simulink model "Main_C0_C3"  (R2023a)
settings: Solver=ode15s  StartTime=0.0  StopTime=1  RelTol=1e-3
model workspace (MAT data in the model file):
  C_IVD = 0.05
  E_IVD1 = 2.1
  E_IVD2 = 2.2
  E_IVD3 = 1.1
  E_IVD4 = 1.7
  E_IVD5 = 3.2
  IVD1 : object (value not decoded)
  IVD2 : object (value not decoded)
  IVD3 : object (value not decoded)
  IVD4 : object (value not decoded)
  IVD5 : object (value not decoded)
  eo_color = [1 0 0]
  io_color = [0 1 0]
  longissimus_color = [1 0 1]
  multifidus_color = [0 1 1]
  muscle_radius = 1
  psoas_color = [0 0 1]
  ra_color = [1 1 0.5]
symbols that are objects in the model workspace (value not decoded): IVD1, IVD2, IVD3, IVD4, IVD5
undefined symbols (not defined in the file or in its folder): AbdFlex, E_TLFflex, IAP_activation_AbdFlex, IAP_Pa, LeftAbdominalMuscleForce, LeftBackMuscleForce, LeftTransverse1MuscleForce, LeftTransverse2MuscleForce, RightAbdominalMuscleForce, RightBackMuscleForce, RightTransverse1MuscleForce, RightTransverse2MuscleForce, TLFflex2, X, Y, Z
libraries: nesl_utility x1235, sm_lib x960, fl_lib x6, simulink_extras x2
(part 7 of 37)

== system Main_C0_C3/TLF Flex ==
  note: F1 - F5 = connectors
      | F6 = right holder
      | F7 = left holder
      | F8 - F10 = right latissimus
      | F11 - F13 = left latissimus
  note: Note: You CAN'T use Fast Restart with Flexible Bodies !
      | They need to be compiled every run, because of E_flex.
  In1 : Inport
  In2 : Inport  Port=2
  Conn L1 : sm_lib/Body Elements/File Solid  ExtGeomFileName=C:\Users\siril\OneDrive\Desktop\TIM-Control\Matlab\Simscape models\Reduced Order Model\CAD\model without nucleus\TLF\L1-conn.step  UnitType=FromFile  ExtGeomFileUnits=m  StepReaderType=HEX  ExportConvexHullGeometry=off  InertiaType=Custom  Mass=1  MassUnits=g  CenterOfMass=[0 0 0]  CenterOfMassUnits=m  MomentsOfInertia=[1 1 1]  MomentsOfInertiaUnits=kg*m^2  ProductsOfInertia=[0 0 0]  ProductsOfInertiaUnits=kg*m^2  BasedOnType=DensityFromFile  Density=1000  DensityUnits=kg/m^3  DoExposeReferenceFrame=off  SerializedFrames=<Frames><Frame><Id>Frame1</Id><Value><Name>to L1_Muscles</Name><Origin><Source>GeometricFeature</Source><FeatureName>point 120</FeatureName></Origin><PrimaryAxis><DefinedDirection>+Z</DefinedDirection><Source>ReferenceFrame</Source><SourceDirection>+Z</SourceDirection><FeatureName></FeatureName></PrimaryAxis><SecondaryAxis><DefinedDirection>+X</DefinedDirection><Source>ReferenceFrame</Source><SourceDirection>+X</SourceDirection><FeatureName></FeatureName></SecondaryAxis></Value></Frame><Frame><Id>Frame2</Id><Value><Name>to TLF</Name><Origin><Source>GeometricFeature</Source><FeatureName>planar surface 1</FeatureName></Origin><PrimaryAxis><DefinedDirection>+Z</DefinedDirection><Source>ReferenceFrame</Source><SourceDirection>+Z</SourceDirection><FeatureName></FeatureName></PrimaryAxis><SecondaryAxis><DefinedDirection>+X</DefinedDirection><Source>ReferenceFrame</Source><SourceDirection>+X</SourceDirection><FeatureName></FeatureName></SecondaryAxis></Value></Frame></Frames>  GraphicType=None  MarkerShape=Sphere  MarkerSize=10  GraphicVisPropType=SimpleVisualProperties  GraphicDiffuseColor=[0.5 0.5 0.5]  GraphicSpecularColor=[0.5 0.5 0.5 1.0]  GraphicAmbientColor=[0.15 0.15 0.15 1.0]  GraphicEmissiveColor=[0.0 0.0 0.0 1.0]  GraphicShininess=75  GraphicOpacity=0.5
  Conn L2 : sm_lib/Body Elements/File Solid  ExtGeomFileName=C:\Users\siril\OneDrive\Desktop\TIM-Control\Matlab\Simscape models\Reduced Order Model\CAD\model without nucleus\TLF\L2-conn.step  UnitType=FromFile  ExtGeomFileUnits=m  StepReaderType=HEX  ExportConvexHullGeometry=off  InertiaType=Custom  Mass=1  MassUnits=g  CenterOfMass=[0 0 0]  CenterOfMassUnits=m  MomentsOfInertia=[1 1 1]  MomentsOfInertiaUnits=kg*m^2  ProductsOfInertia=[0 0 0]  ProductsOfInertiaUnits=kg*m^2  BasedOnType=DensityFromFile  Density=1000  DensityUnits=kg/m^3  DoExposeReferenceFrame=off  SerializedFrames=<Frames><Frame><Id>Frame1</Id><Value><Name>to Muscles L2</Name><Origin><Source>GeometricFeature</Source><FeatureName>point 118</FeatureName></Origin><PrimaryAxis><DefinedDirection>+Z</DefinedDirection><Source>ReferenceFrame</Source><SourceDirection>+Z</SourceDirection><FeatureName></FeatureName></PrimaryAxis><SecondaryAxis><DefinedDirection>+X</DefinedDirection><Source>ReferenceFrame</Source><SourceDirection>+X</SourceDirection><FeatureName></FeatureName></SecondaryAxis></Value></Frame><Frame><Id>Frame2</Id><Value><Name>to TLF</Name><Origin><Source>GeometricFeature</Source><FeatureName>planar surface 1</FeatureName></Origin><PrimaryAxis><DefinedDirection>+Z</DefinedDirection><Source>ReferenceFrame</Source><SourceDirection>+Z</SourceDirection><FeatureName></FeatureName></PrimaryAxis><SecondaryAxis><DefinedDirection>+X</DefinedDirection><Source>ReferenceFrame</Source><SourceDirection>+X</SourceDirection><FeatureName></FeatureName></SecondaryAxis></Value></Frame></Frames>  GraphicType=None  MarkerShape=Sphere  MarkerSize=10  GraphicVisPropType=SimpleVisualProperties  GraphicDiffuseColor=[0.5 0.5 0.5]  GraphicSpecularColor=[0.5 0.5 0.5 1.0]  GraphicAmbientColor=[0.15 0.15 0.15 1.0]  GraphicEmissiveColor=[0.0 0.0 0.0 1.0]  GraphicShininess=75  GraphicOpacity=0.5
  Conn L3 : sm_lib/Body Elements/File Solid  ExtGeomFileName=C:\Users\siril\OneDrive\Desktop\TIM-Control\Matlab\Simscape models\Reduced Order Model\CAD\model without nucleus\TLF\L3-conn.step  UnitType=FromFile  ExtGeomFileUnits=m  StepReaderType=HEX  ExportConvexHullGeometry=off  InertiaType=Custom  Mass=1  MassUnits=g  CenterOfMass=[0 0 0]  CenterOfMassUnits=m  MomentsOfInertia=[1 1 1]  MomentsOfInertiaUnits=kg*m^2  ProductsOfInertia=[0 0 0]  ProductsOfInertiaUnits=kg*m^2  BasedOnType=DensityFromFile  Density=1000  DensityUnits=kg/m^3  DoExposeReferenceFrame=off  SerializedFrames=<Frames><Frame><Id>Frame1</Id><Value><Name>to Muscles L3</Name><Origin><Source>GeometricFeature</Source><FeatureName>point 147</FeatureName></Origin><PrimaryAxis><DefinedDirection>+Z</DefinedDirection><Source>ReferenceFrame</Source><SourceDirection>+Z</SourceDirection><FeatureName></FeatureName></PrimaryAxis><SecondaryAxis><DefinedDirection>+X</DefinedDirection><Source>ReferenceFrame</Source><SourceDirection>+X</SourceDirection><FeatureName></FeatureName></SecondaryAxis></Value></Frame><Frame><Id>Frame2</Id><Value><Name>to TLF</Name><Origin><Source>GeometricFeature</Source><FeatureName>planar surface 1</FeatureName></Origin><PrimaryAxis><DefinedDirection>+Z</DefinedDirection><Source>ReferenceFrame</Source><SourceDirection>+Z</SourceDirection><FeatureName></FeatureName></PrimaryAxis><SecondaryAxis><DefinedDirection>+X</DefinedDirection><Source>ReferenceFrame</Source><SourceDirection>+X</SourceDirection><FeatureName></FeatureName></SecondaryAxis></Value></Frame></Frames>  GraphicType=None  MarkerShape=Sphere  MarkerSize=10  GraphicVisPropType=SimpleVisualProperties  GraphicDiffuseColor=[0.5 0.5 0.5]  GraphicSpecularColor=[0.5 0.5 0.5 1.0]  GraphicAmbientColor=[0.15 0.15 0.15 1.0]  GraphicEmissiveColor=[0.0 0.0 0.0 1.0]  GraphicShininess=75  GraphicOpacity=0.5
  Conn L4 : sm_lib/Body Elements/File Solid  ExtGeomFileName=C:\Users\siril\OneDrive\Desktop\TIM-Control\Matlab\Simscape models\Reduced Order Model\CAD\model without nucleus\TLF\L4-conn.step  UnitType=FromFile  ExtGeomFileUnits=m  StepReaderType=HEX  ExportConvexHullGeometry=off  InertiaType=Custom  Mass=1  MassUnits=g  CenterOfMass=[0 0 0]  CenterOfMassUnits=m  MomentsOfInertia=[1 1 1]  MomentsOfInertiaUnits=kg*m^2  ProductsOfInertia=[0 0 0]  ProductsOfInertiaUnits=kg*m^2  BasedOnType=DensityFromFile  Density=1000  DensityUnits=kg/m^3  DoExposeReferenceFrame=off  SerializedFrames=<Frames><Frame><Id>Frame1</Id><Value><Name>to Muscles L4</Name><Origin><Source>GeometricFeature</Source><FeatureName>point 96</FeatureName></Origin><PrimaryAxis><DefinedDirection>+Z</DefinedDirection><Source>ReferenceFrame</Source><SourceDirection>+Z</SourceDirection><FeatureName></FeatureName></PrimaryAxis><SecondaryAxis><DefinedDirection>+X</DefinedDirection><Source>ReferenceFrame</Source><SourceDirection>+X</SourceDirection><FeatureName></FeatureName></SecondaryAxis></Value></Frame><Frame><Id>Frame2</Id><Value><Name>to TLF</Name><Origin><Source>GeometricFeature</Source><FeatureName>planar surface 3</FeatureName></Origin><PrimaryAxis><DefinedDirection>+Z</DefinedDirection><Source>ReferenceFrame</Source><SourceDirection>+Z</SourceDirection><FeatureName></FeatureName></PrimaryAxis><SecondaryAxis><DefinedDirection>+X</DefinedDirection><Source>ReferenceFrame</Source><SourceDirection>+X</SourceDirection><FeatureName></FeatureName></SecondaryAxis></Value></Frame></Frames>  GraphicType=None  MarkerShape=Sphere  MarkerSize=10  GraphicVisPropType=SimpleVisualProperties  GraphicDiffuseColor=[0.5 0.5 0.5]  GraphicSpecularColor=[0.5 0.5 0.5 1.0]  GraphicAmbientColor=[0.15 0.15 0.15 1.0]  GraphicEmissiveColor=[0.0 0.0 0.0 1.0]  GraphicShininess=75  GraphicOpacity=0.5
  Conn L5 : sm_lib/Body Elements/File Solid  ExtGeomFileName=C:\Users\siril\OneDrive\Desktop\TIM-Control\Matlab\Simscape models\Reduced Order Model\CAD\model without nucleus\TLF\L5-conn.step  UnitType=FromFile  ExtGeomFileUnits=m  StepReaderType=HEX  ExportConvexHullGeometry=off  InertiaType=Custom  Mass=1  MassUnits=g  CenterOfMass=[0 0 0]  CenterOfMassUnits=m  MomentsOfInertia=[1 1 1]  MomentsOfInertiaUnits=kg*m^2  ProductsOfInertia=[0 0 0]  ProductsOfInertiaUnits=kg*m^2  BasedOnType=DensityFromFile  Density=1000  DensityUnits=kg/m^3  DoExposeReferenceFrame=off  SerializedFrames=<Frames><Frame><Id>Frame1</Id><Value><Name>to Muscles L5</Name><Origin><Source>GeometricFeature</Source><FeatureName>point 125</FeatureName></Origin><PrimaryAxis><DefinedDirection>+Z</DefinedDirection><Source>ReferenceFrame</Source><SourceDirection>+Z</SourceDirection><FeatureName></FeatureName></PrimaryAxis><SecondaryAxis><DefinedDirection>+X</DefinedDirection><Source>ReferenceFrame</Source><SourceDirection>+X</SourceDirection><FeatureName></FeatureName></SecondaryAxis></Value></Frame><Frame><Id>Frame2</Id><Value><Name>to TLF</Name><Origin><Source>GeometricFeature</Source><FeatureName>planar surface 1</FeatureName></Origin><PrimaryAxis><DefinedDirection>+Z</DefinedDirection><Source>ReferenceFrame</Source><SourceDirection>+Z</SourceDirection><FeatureName></FeatureName></PrimaryAxis><SecondaryAxis><DefinedDirection>+X</DefinedDirection><Source>ReferenceFrame</Source><SourceDirection>+X</SourceDirection><FeatureName></FeatureName></SecondaryAxis></Value></Frame></Frames>  GraphicType=None  MarkerShape=Sphere  MarkerSize=10  GraphicVisPropType=SimpleVisualProperties  GraphicDiffuseColor=[0.5 0.5 0.5]  GraphicSpecularColor=[0.5 0.5 0.5 1.0]  GraphicAmbientColor=[0.15 0.15 0.15 1.0]  GraphicEmissiveColor=[0.0 0.0 0.0 1.0]  GraphicShininess=75  GraphicOpacity=0.5
  Holder left : sm_lib/Body Elements/File Solid  ExtGeomFileName=C:\Users\siril\OneDrive\Desktop\TIM-Control\Matlab\Simscape models\Reduced Order Model\CAD\model without nucleus\TLF\Holder_left.step  UnitType=FromFile  ExtGeomFileUnits=m  StepReaderType=HEX  ExportConvexHullGeometry=off  InertiaType=Custom  Mass=1  MassUnits=g  CenterOfMass=[0 0 0]  CenterOfMassUnits=m  MomentsOfInertia=[1 1 1]  MomentsOfInertiaUnits=kg*m^2  ProductsOfInertia=[0 0 0]  ProductsOfInertiaUnits=kg*m^2  BasedOnType=DensityFromFile  Density=1000  DensityUnits=kg/m^3  DoExposeReferenceFrame=on  SerializedFrames=<Frames><Frame><Id>Frame1</Id><Value><Name>F1</Name><Origin><Source>GeometricFeature</Source><FeatureName>general surface 1</FeatureName></Origin><PrimaryAxis><DefinedDirection>+Z</DefinedDirection><Source>ReferenceFrame</Source><SourceDirection>+Z</SourceDirection><FeatureName></FeatureName></PrimaryAxis><SecondaryAxis><DefinedDirection>+X</DefinedDirection><Source>ReferenceFrame</Source><SourceDirection>+X</SourceDirection><FeatureName></FeatureName></SecondaryAxis></Value></Frame></Frames>  GraphicType=None  MarkerShape=Sphere  MarkerSize=10  GraphicVisPropType=SimpleVisualProperties  GraphicDiffuseColor=[0.5 0.5 0.5]  GraphicSpecularColor=[0.5 0.5 0.5 1.0]  GraphicAmbientColor=[0.15 0.15 0.15 1.0]  GraphicEmissiveColor=[0.0 0.0 0.0 1.0]  GraphicShininess=75  GraphicOpacity=1.0
  Holder right : sm_lib/Body Elements/File Solid  ExtGeomFileName=C:\Users\siril\OneDrive\Desktop\TIM-Control\Matlab\Simscape models\Reduced Order Model\CAD\model without nucleus\TLF\Holder_right.step  UnitType=FromFile  ExtGeomFileUnits=m  StepReaderType=HEX  ExportConvexHullGeometry=off  InertiaType=Custom  Mass=1  MassUnits=g  CenterOfMass=[0 0 0]  CenterOfMassUnits=m  MomentsOfInertia=[1 1 1]  MomentsOfInertiaUnits=kg*m^2  ProductsOfInertia=[0 0 0]  ProductsOfInertiaUnits=kg*m^2  BasedOnType=DensityFromFile  Density=1000  DensityUnits=kg/m^3  DoExposeReferenceFrame=on  SerializedFrames=<Frames><Frame><Id>Frame1</Id><Value><Name>F1</Name><Origin><Source>GeometricFeature</Source><FeatureName>general surface 1</FeatureName></Origin><PrimaryAxis><DefinedDirection>+Z</DefinedDirection><Source>ReferenceFrame</Source><SourceDirection>+Z</SourceDirection><FeatureName></FeatureName></PrimaryAxis><SecondaryAxis><DefinedDirection>+X</DefinedDirection><Source>ReferenceFrame</Source><SourceDirection>+X</SourceDirection><FeatureName></FeatureName></SecondaryAxis></Value></Frame></Frames>  GraphicType=None  MarkerShape=Sphere  MarkerSize=10  GraphicVisPropType=SimpleVisualProperties  GraphicDiffuseColor=[0.5 0.5 0.5]  GraphicSpecularColor=[0.5 0.5 0.5 1.0]  GraphicAmbientColor=[0.15 0.15 0.15 1.0]  GraphicEmissiveColor=[0.0 0.0 0.0 1.0]  GraphicShininess=75  GraphicOpacity=1.0
  Latissimus Dorsi : Subsystem
  TLF_Flex : sm_lib/Body Elements/Flexible Bodies/Reduced Order Flexible Solid  GraphicAmbientColor=[0.15 0.15 0.15 1.0]  GraphicDiffuseColor=[0.07451 0.6235 1]  DampingType=Proportional  GraphicEmissiveColor=[0.0 0.0 0.0 1.0]  GraphicFacetVertexIndices=TLFflex2.GraphicFacetVertexIndices  InterfaceFrameOrientations=TLFflex2.InterfaceFrameOrientations  GraphicType=DeformedGeometry  MassMatrix=TLFflex2.MassMatrix  NumRetainedModes=1  NumberOfInterfaceFrames=13  GraphicOpacity=0.2  GraphicReconstructionMatrix=TLFflex2.GraphicReconstructionMatrix  ReductionType=None  InterfaceFrameOrigins=TLFflex2.InterfaceFrameOrigins  GraphicShininess=75  GraphicSpecularColor=[0.5 0.5 0.5 1.0]  StiffnessMatrix=TLFflex2.StiffnessMatrix * E_TLFflex  GeomUnitType=FromFile  GraphicVertexCoordinates=TLFflex2.GraphicVertexCoordinates  VisRecursionLimit=3  GraphicVisPropType=SimpleVisualProperties  LengthUnit=m  MassUnit=kg  TimeUnit=s  UnitSystemType=SI  ProportionalDampingAlpha=0  ProportionalDampingBeta=0.05  UniformModalDampingRatio=0.01  DampingMatrix=[]
  Weld Joint11 : sm_lib/Joints/Weld Joint  JointMode=Normal  SenseConstraintForce=off  SenseConstraintForceX=off  SenseConstraintForceY=off  SenseConstraintForceZ=off  SenseConstraintTorque=off  SenseConstraintTorqueX=off  SenseConstraintTorqueY=off  SenseConstraintTorqueZ=off  SenseTotalForce=off  SenseTotalForceX=off  SenseTotalForceY=off  SenseTotalForceZ=off  SenseTotalTorque=off  SenseTotalTorqueX=off  SenseTotalTorqueY=off  SenseTotalTorqueZ=off  CompositeWrenchDir=FollowerOnBase  CompositeWrenchFrame=BaseFrame
  Weld Joint12 : sm_lib/Joints/Weld Joint  JointMode=Normal  SenseConstraintForce=off  SenseConstraintForceX=off  SenseConstraintForceY=off  SenseConstraintForceZ=off  SenseConstraintTorque=off  SenseConstraintTorqueX=off  SenseConstraintTorqueY=off  SenseConstraintTorqueZ=off  SenseTotalForce=off  SenseTotalForceX=off  SenseTotalForceY=off  SenseTotalForceZ=off  SenseTotalTorque=off  SenseTotalTorqueX=off  SenseTotalTorqueY=off  SenseTotalTorqueZ=off  CompositeWrenchDir=FollowerOnBase  CompositeWrenchFrame=BaseFrame
  Conn1 : PMIOPort  Side=Left
  Conn2 : PMIOPort  Port=2  Side=Left
  Conn3 : PMIOPort  Port=3  Side=Left
  Conn4 : PMIOPort  Port=4  Side=Left
  Conn5 : PMIOPort  Port=5  Side=Left
  Conn6 : PMIOPort  Port=6  Side=Right
  Wrap1 : PMIOPort  Port=7  Side=Right
  Wrap2 : PMIOPort  Port=8  Side=Right
  Conn9 : PMIOPort  Port=9  Side=Left
  Conn10 : PMIOPort  Port=10  Side=Right
  Conn11 : PMIOPort  Port=11  Side=Left
  Conn12 : PMIOPort  Port=12  Side=Left
  Conn13 : PMIOPort  Port=13  Side=Right
  Wrap3 : PMIOPort  Port=14  Side=Right
  Conn15 : PMIOPort  Port=15  Side=Left
  Wrap4 : PMIOPort  Port=16  Side=Right
  Conn17 : PMIOPort  Port=17  Side=Left
  Wrap5 : PMIOPort  Port=18  Side=Right
  wires:
  In1/1 -> Latissimus Dorsi/1(In1)
  In2/1 -> Latissimus Dorsi/2(In2)
  connections:
  Latissimus Dorsi/LConn5 -- Conn17/RConn1
  Latissimus Dorsi/RConn10 -- Wrap5/RConn1
  Latissimus Dorsi/LConn6 -- Conn9/RConn1
  Conn5/RConn1 -- Conn L2/LConn1
  Conn13/RConn1 -- Latissimus Dorsi/RConn1
  Latissimus Dorsi/LConn4 -- Conn15/RConn1
  Conn4/RConn1 -- Conn L5/LConn1
  Conn1/RConn1 -- Conn L4/LConn1
  Latissimus Dorsi/RConn6 -- Wrap2/RConn1
  Latissimus Dorsi/RConn8 -- Wrap3/RConn1
  Latissimus Dorsi/RConn7 -- Conn10/RConn1
  Conn6/RConn1 -- Latissimus Dorsi/RConn11
  Latissimus Dorsi/RConn5 -- Wrap1/RConn1
  Weld Joint11/RConn1 -- TLF_Flex/RConn3
  Holder right/LConn1 -- Weld Joint11/LConn1
  Conn2/RConn1 -- Conn L3/LConn1
  Conn L4/RConn1 -- TLF_Flex/RConn2
  Holder left/LConn1 -- Weld Joint12/LConn1
  Weld Joint12/RConn1 -- TLF_Flex/LConn4
  Latissimus Dorsi/LConn7 -- Conn11/RConn1
  Latissimus Dorsi/RConn9 -- Wrap4/RConn1
  Latissimus Dorsi/RConn2 -- TLF_Flex/LConn5
  Latissimus Dorsi/LConn1 -- TLF_Flex/RConn4
  Latissimus Dorsi/LConn3 -- TLF_Flex/RConn6
  Latissimus Dorsi/RConn4 -- TLF_Flex/LConn7
  Conn3/RConn1 -- Conn L1/LConn1
  Holder right/RConn1 -- Conn12/RConn1 -- Holder left/RConn1
  Conn L1/RConn1 -- TLF_Flex/LConn1
  Latissimus Dorsi/RConn3 -- TLF_Flex/LConn6
  Conn L3/RConn1 -- TLF_Flex/LConn2
  Latissimus Dorsi/LConn2 -- TLF_Flex/RConn5
  Conn L5/RConn1 -- TLF_Flex/LConn3
  Conn L2/RConn1 -- TLF_Flex/RConn1

== system Main_C0_C3/Interspinous Ligaments/ISL Visualization ==
  Ligament1 : Subsystem
  Ligament2 : Subsystem
  Ligament3 : Subsystem
  Ligament4 : Subsystem
  Ligament5 : Subsystem
  MuscleEnd2 : PMIOPort  Side=Right
  MuscleEnd1 : PMIOPort  Port=2  Side=Right
  MuscleEnd3 : PMIOPort  Port=3  Side=Right
  MuscleEnd4 : PMIOPort  Port=4  Side=Right
  MuscleEnd5 : PMIOPort  Port=5  Side=Right
  MuscleEnd6 : PMIOPort  Port=6  Side=Right
  MuscleEnd7 : PMIOPort  Port=7  Side=Right
  MuscleEnd8 : PMIOPort  Port=8  Side=Right
  MuscleEnd9 : PMIOPort  Port=9  Side=Right
  MuscleEnd10 : PMIOPort  Port=10  Side=Right
  R : PMIOPort  Port=11  Side=Left
  connections:
  Ligament2/RConn2 -- MuscleEnd6/RConn1
  Ligament4/RConn2 -- MuscleEnd1/RConn1
  Ligament5/RConn1 -- MuscleEnd3/RConn1
  Ligament2/RConn1 -- MuscleEnd9/RConn1
  Ligament5/RConn2 -- MuscleEnd2/RConn1
  Ligament1/RConn2 -- MuscleEnd10/RConn1
  Ligament3/RConn1 -- MuscleEnd7/RConn1
  Ligament3/RConn2 -- MuscleEnd5/RConn1
  Ligament4/RConn3 -- Ligament3/RConn3 -- Ligament2/RConn3 -- R/RConn1 -- Ligament1/RConn3 -- Ligament5/RConn3
  Ligament4/RConn1 -- MuscleEnd4/RConn1
  Ligament1/RConn1 -- MuscleEnd8/RConn1

== system Main_C0_C3/Interspinous Ligaments/Visualization ==
  Belt-Cable Properties{1..4,55} (5 alike) : sm_lib/Belts and Cables/Belt-Cable Properties  DrumBeltCableAlignment=Unrestricted  GraphicType=PitchLine  GraphicVisPropType=SimpleVisualProperties  GraphicDiffuseColor=[1 0 1]  GraphicSpecularColor=[0.5 0.5 0.5 1.0]  GraphicAmbientColor=[0.15 0.15 0.15 1.0]  GraphicEmissiveColor=[0.0 0.0 0.0 1.0]  GraphicShininess=75  GraphicOpacity=1.0
  Belt-Cable End{1..8,110..111} (10 alike) : sm_lib/Belts and Cables/Belt-Cable End
  Conn1 : PMIOPort  Side=Left
  Conn2 : PMIOPort  Port=2  Side=Left
  Conn3 : PMIOPort  Port=3  Side=Left
  Conn4 : PMIOPort  Port=4  Side=Left
  Conn5 : PMIOPort  Port=5  Side=Left
  Conn6 : PMIOPort  Port=6  Side=Left
  Conn7 : PMIOPort  Port=7  Side=Left
  Conn8 : PMIOPort  Port=8  Side=Left
  Conn9 : PMIOPort  Port=9  Side=Left
  Conn10 : PMIOPort  Port=10  Side=Left
  connections:
  Belt-Cable End8/LConn1 -- Conn6/RConn1
  Belt-Cable End3/LConn1 -- Conn1/RConn1
  Belt-Cable End7/LConn1 -- Conn2/RConn1
  Belt-Cable End5/LConn1 -- Conn8/RConn1
  Belt-Cable End2/LConn1 -- Conn9/RConn1
  Belt-Cable End1/LConn1 -- Conn5/RConn1
  Belt-Cable End110/LConn1 -- Conn4/RConn1
  Belt-Cable End2/RConn1 -- Belt-Cable End1/RConn1 -- Belt-Cable Properties1/LConn1
  Belt-Cable End111/RConn1 -- Belt-Cable End110/RConn1 -- Belt-Cable Properties55/LConn1
  Belt-Cable End111/LConn1 -- Conn10/RConn1
  Belt-Cable End5/RConn1 -- Belt-Cable End4/RConn1 -- Belt-Cable Properties3/LConn1
  Belt-Cable End8/RConn1 -- Belt-Cable End7/RConn1 -- Belt-Cable Properties4/LConn1
  Belt-Cable End4/LConn1 -- Conn3/RConn1
  Belt-Cable End6/LConn1 -- Conn7/RConn1
  Belt-Cable End6/RConn1 -- Belt-Cable End3/RConn1 -- Belt-Cable Properties2/LConn1

== system Main_C0_C3/Left and Right Intertransverse Ligaments/ITL Visualization - debug ==
  Ligament1 : Subsystem
  Ligament10 : Subsystem
  Ligament2 : Subsystem
  Ligament3 : Subsystem
  Ligament4 : Subsystem
  Ligament5 : Subsystem
  Ligament6 : Subsystem
  Ligament7 : Subsystem
  Ligament8 : Subsystem
  Ligament9 : Subsystem
  MuscleEnd2 : PMIOPort  Side=Right
  MuscleEnd1 : PMIOPort  Port=2  Side=Right
  MuscleEnd3 : PMIOPort  Port=3  Side=Right
  MuscleEnd4 : PMIOPort  Port=4  Side=Right
  MuscleEnd5 : PMIOPort  Port=5  Side=Right
  MuscleEnd6 : PMIOPort  Port=6  Side=Right
  MuscleEnd7 : PMIOPort  Port=7  Side=Right
  MuscleEnd8 : PMIOPort  Port=8  Side=Right
  MuscleEnd9 : PMIOPort  Port=9  Side=Right
  MuscleEnd10 : PMIOPort  Port=10  Side=Right
  R : PMIOPort  Port=11  Side=Left
  MuscleEnd11 : PMIOPort  Port=12  Side=Right
  MuscleEnd12 : PMIOPort  Port=13  Side=Right
  MuscleEnd13 : PMIOPort  Port=14  Side=Right
  MuscleEnd14 : PMIOPort  Port=15  Side=Right
  MuscleEnd15 : PMIOPort  Port=16  Side=Right
  MuscleEnd16 : PMIOPort  Port=17  Side=Right
  MuscleEnd17 : PMIOPort  Port=18  Side=Right
  MuscleEnd18 : PMIOPort  Port=19  Side=Right
  MuscleEnd19 : PMIOPort  Port=20  Side=Right
  MuscleEnd20 : PMIOPort  Port=21  Side=Right
  connections:
  Ligament9/RConn1 -- MuscleEnd10/RConn1
  Ligament9/RConn2 -- MuscleEnd9/RConn1
  Ligament8/RConn2 -- MuscleEnd6/RConn1
  Ligament7/RConn1 -- MuscleEnd5/RConn1
  Ligament5/RConn1 -- MuscleEnd17/RConn1
  Ligament2/RConn2 -- MuscleEnd16/RConn1
  Ligament10/RConn2 -- MuscleEnd4/RConn1
  Ligament10/RConn1 -- MuscleEnd7/RConn1
  Ligament6/RConn2 -- MuscleEnd2/RConn1
  Ligament1/RConn1 -- MuscleEnd15/RConn1
  Ligament2/RConn1 -- MuscleEnd18/RConn1
  Ligament4/RConn1 -- MuscleEnd20/RConn1
  Ligament8/RConn1 -- MuscleEnd8/RConn1
  Ligament3/RConn1 -- MuscleEnd12/RConn1
  Ligament5/RConn2 -- MuscleEnd14/RConn1
  Ligament4/RConn2 -- MuscleEnd19/RConn1
  Ligament7/RConn2 -- MuscleEnd3/RConn1
  Ligament1/RConn2 -- MuscleEnd13/RConn1
  Ligament6/RConn1 -- MuscleEnd1/RConn1
  Ligament3/RConn2 -- MuscleEnd11/RConn1
  R/RConn1 -- Ligament2/RConn3 -- Ligament4/RConn3 -- Ligament5/RConn3 -- Ligament1/RConn3 -- Ligament6/RConn3 -- Ligament7/RConn3 -- Ligament8/RConn3 -- Ligament10/RConn3 -- Ligament9/RConn3 -- Ligament3/RConn3

== system Main_C0_C3/Left and Right Intertransverse Ligaments/Rope Visualization ==
  Belt-Cable Properties{1..10} (10 alike) : sm_lib/Belts and Cables/Belt-Cable Properties  DrumBeltCableAlignment=Unrestricted  GraphicType=PitchLine  GraphicVisPropType=SimpleVisualProperties  GraphicDiffuseColor=[0 0 1]  GraphicSpecularColor=[0.5 0.5 0.5 1.0]  GraphicAmbientColor=[0.15 0.15 0.15 1.0]  GraphicEmissiveColor=[0.0 0.0 0.0 1.0]  GraphicShininess=75  GraphicOpacity=1.0
  Belt-Cable End{1..20} (20 alike) : sm_lib/Belts and Cables/Belt-Cable End
  Conn1 : PMIOPort  Side=Left
  Conn2 : PMIOPort  Port=2  Side=Left
  Conn3 : PMIOPort  Port=3  Side=Left
  Conn4 : PMIOPort  Port=4  Side=Left
  Conn5 : PMIOPort  Port=5  Side=Left
  Conn6 : PMIOPort  Port=6  Side=Left
  Conn7 : PMIOPort  Port=7  Side=Left
  Conn8 : PMIOPort  Port=8  Side=Left
  Conn9 : PMIOPort  Port=9  Side=Left
  Conn10 : PMIOPort  Port=10  Side=Left
  Conn11 : PMIOPort  Port=11  Side=Left
  Conn12 : PMIOPort  Port=12  Side=Left
  Conn13 : PMIOPort  Port=13  Side=Left
  Conn14 : PMIOPort  Port=14  Side=Left
  Conn15 : PMIOPort  Port=15  Side=Left
  Conn16 : PMIOPort  Port=16  Side=Left
  Conn17 : PMIOPort  Port=17  Side=Left
  Conn18 : PMIOPort  Port=18  Side=Left
  Conn19 : PMIOPort  Port=19  Side=Left
  Conn20 : PMIOPort  Port=20  Side=Left
  connections:
  Belt-Cable End12/LConn1 -- Conn20/RConn1
  Belt-Cable End16/LConn1 -- Conn15/RConn1
  Belt-Cable End20/LConn1 -- Conn13/RConn1
  Belt-Cable End4/LConn1 -- Conn8/RConn1
  Belt-Cable End13/LConn1 -- Conn18/RConn1
  Belt-Cable End15/LConn1 -- Conn17/RConn1
  Belt-Cable End19/LConn1 -- Conn16/RConn1
  Belt-Cable End10/LConn1 -- Conn10/RConn1
  Belt-Cable End11/LConn1 -- Conn12/RConn1
  Belt-Cable End8/LConn1 -- Conn1/RConn1
  Belt-Cable End1/LConn1 -- Conn6/RConn1
  Belt-Cable End9/RConn1 -- Belt-Cable End10/RConn1 -- Belt-Cable Properties5/LConn1
  Belt-Cable End6/LConn1 -- Conn9/RConn1
  Belt-Cable End5/LConn1 -- Conn3/RConn1
  Belt-Cable End14/LConn1 -- Conn14/RConn1
  Belt-Cable End2/LConn1 -- Conn7/RConn1
  Belt-Cable End3/LConn1 -- Conn4/RConn1
  Belt-Cable End15/RConn1 -- Belt-Cable End14/RConn1 -- Belt-Cable Properties7/LConn1
  Belt-Cable End17/LConn1 -- Conn19/RConn1
  Belt-Cable End19/RConn1 -- Belt-Cable End18/RConn1 -- Belt-Cable Properties9/LConn1
  Belt-Cable End5/RConn1 -- Belt-Cable End6/RConn1 -- Belt-Cable Properties3/LConn1
  Belt-Cable End13/RConn1 -- Belt-Cable Properties6/LConn1 -- Belt-Cable End11/RConn1
  Belt-Cable End9/LConn1 -- Conn5/RConn1
  Belt-Cable End12/RConn1 -- Belt-Cable End20/RConn1 -- Belt-Cable Properties10/LConn1
  Belt-Cable End4/RConn1 -- Belt-Cable End3/RConn1 -- Belt-Cable Properties2/LConn1
  Belt-Cable End7/LConn1 -- Conn2/RConn1
  Belt-Cable End7/RConn1 -- Belt-Cable End8/RConn1 -- Belt-Cable Properties4/LConn1
  Belt-Cable End18/LConn1 -- Conn11/RConn1
  Belt-Cable End17/RConn1 -- Belt-Cable End16/RConn1 -- Belt-Cable Properties8/LConn1
  Belt-Cable End1/RConn1 -- Belt-Cable End2/RConn1 -- Belt-Cable Properties1/LConn1

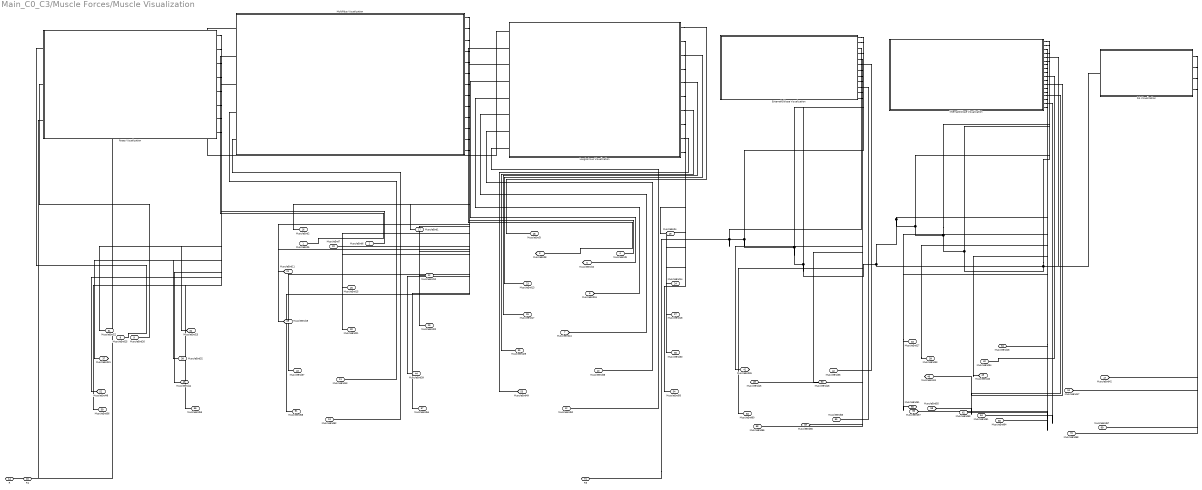
== system Main_C0_C3/Muscle Forces/Muscle Visualization ==
  ExternalOblique Visualization : Subsystem
  InternalOblique Visualization : Subsystem
  Longissimus Visualization : Subsystem
  Multifidus Visualization : Subsystem
  Psoas Visualization : Subsystem
  RA Visualization : Subsystem
  MuscleEnd5 : PMIOPort  Side=Left
  MuscleEnd6 : PMIOPort  Port=2  Side=Left
  MuscleEnd8 : PMIOPort  Port=3  Side=Left
  MuscleEnd9 : PMIOPort  Port=4  Side=Left
  MuscleEnd10 : PMIOPort  Port=5  Side=Left
  MuscleEnd16 : PMIOPort  Port=6  Side=Left
  MuscleEnd24 : PMIOPort  Port=7  Side=Left
  MuscleEnd25 : PMIOPort  Port=8  Side=Left
  MuscleEnd26 : PMIOPort  Port=9  Side=Left
  MuscleEnd38 : PMIOPort  Port=10  Side=Left
  MuscleEnd43 : PMIOPort  Port=11  Side=Left
  MuscleEnd52 : PMIOPort  Port=12  Side=Left
  MuscleEnd62 : PMIOPort  Port=13  Side=Left
  R : PMIOPort  Port=14  Side=Left
  R1 : PMIOPort  Port=15  Side=Left
  MuscleEnd2 : PMIOPort  Port=16  Side=Right
  MuscleEnd1 : PMIOPort  Port=17  Side=Right
  MuscleEnd3 : PMIOPort  Port=18  Side=Right
  MuscleEnd4 : PMIOPort  Port=19  Side=Right
  MuscleEnd7 : PMIOPort  Port=20  Side=Right
  MuscleEnd11 : PMIOPort  Port=21  Side=Right
  MuscleEnd12 : PMIOPort  Port=22  Side=Right
  MuscleEnd13 : PMIOPort  Port=23  Side=Right
  MuscleEnd14 : PMIOPort  Port=24  Side=Right
  MuscleEnd15 : PMIOPort  Port=25  Side=Right
  MuscleEnd17 : PMIOPort  Port=26  Side=Right
  MuscleEnd18 : PMIOPort  Port=27  Side=Right
  MuscleEnd19 : PMIOPort  Port=28  Side=Right
  MuscleEnd20 : PMIOPort  Port=29  Side=Right
  MuscleEnd21 : PMIOPort  Port=30  Side=Right
  MuscleEnd22 : PMIOPort  Port=31  Side=Right
  MuscleEnd23 : PMIOPort  Port=32  Side=Right
  MuscleEnd27 : PMIOPort  Port=33  Side=Right
  MuscleEnd28 : PMIOPort  Port=34  Side=Right
  MuscleEnd29 : PMIOPort  Port=35  Side=Right
  MuscleEnd30 : PMIOPort  Port=36  Side=Right
  MuscleEnd31 : PMIOPort  Port=37  Side=Right
  MuscleEnd32 : PMIOPort  Port=38  Side=Right
  MuscleEnd33 : PMIOPort  Port=39  Side=Right
  MuscleEnd34 : PMIOPort  Port=40  Side=Right
  MuscleEnd35 : PMIOPort  Port=41  Side=Right
  MuscleEnd36 : PMIOPort  Port=42  Side=Right
  MuscleEnd37 : PMIOPort  Port=43  Side=Right
  MuscleEnd39 : PMIOPort  Port=44  Side=Right
  MuscleEnd40 : PMIOPort  Port=45  Side=Right
  MuscleEnd41 : PMIOPort  Port=46  Side=Right
  MuscleEnd42 : PMIOPort  Port=47  Side=Right
  MuscleEnd44 : PMIOPort  Port=48  Side=Right
  MuscleEnd45 : PMIOPort  Port=49  Side=Right
  MuscleEnd46 : PMIOPort  Port=50  Side=Right
  MuscleEnd47 : PMIOPort  Port=51  Side=Right
  MuscleEnd48 : PMIOPort  Port=52  Side=Right
  MuscleEnd49 : PMIOPort  Port=53  Side=Right
  MuscleEnd50 : PMIOPort  Port=54  Side=Right
  MuscleEnd51 : PMIOPort  Port=55  Side=Right
  MuscleEnd53 : PMIOPort  Port=56  Side=Right
  MuscleEnd54 : PMIOPort  Port=57  Side=Right
  MuscleEnd55 : PMIOPort  Port=58  Side=Right
  MuscleEnd56 : PMIOPort  Port=59  Side=Right
  MuscleEnd57 : PMIOPort  Port=60  Side=Right
  MuscleEnd58 : PMIOPort  Port=61  Side=Right
  MuscleEnd59 : PMIOPort  Port=62  Side=Right
  MuscleEnd60 : PMIOPort  Port=63  Side=Right
  MuscleEnd61 : PMIOPort  Port=64  Side=Right
  MuscleEnd63 : PMIOPort  Port=65  Side=Right
  MuscleEnd64 : PMIOPort  Port=66  Side=Right
  MuscleEnd65 : PMIOPort  Port=67  Side=Right
  MuscleEnd66 : PMIOPort  Port=68  Side=Right
  MuscleEnd67 : PMIOPort  Port=69  Side=Right
  MuscleEnd68 : PMIOPort  Port=70  Side=Right
  R5 : PMIOPort  Port=71  Side=Right
  connections:
  InternalOblique Visualization/RConn11 -- MuscleEnd40/RConn1
  InternalOblique Visualization/RConn15 -- MuscleEnd55/RConn1
  InternalOblique Visualization/RConn8 -- MuscleEnd28/RConn1
  InternalOblique Visualization/RConn12 -- MuscleEnd41/RConn1
  InternalOblique Visualization/RConn18 -- MuscleEnd64/RConn1
  InternalOblique Visualization/RConn9 -- MuscleEnd33/RConn1
  Multifidus Visualization/RConn11 -- MuscleEnd39/RConn1
  Multifidus Visualization/RConn10 -- MuscleEnd37/RConn1
  Multifidus Visualization/LConn5 -- MuscleEnd62/RConn1
  Multifidus Visualization/RConn6 -- MuscleEnd15/RConn1
  Multifidus Visualization/LConn2 -- MuscleEnd5/RConn1
  Multifidus Visualization/RConn9 -- MuscleEnd21/RConn1
  Multifidus Visualization/RConn2 -- MuscleEnd1/RConn1
  InternalOblique Visualization/RConn16 -- MuscleEnd59/RConn1
  Multifidus Visualization/RConn1 -- MuscleEnd2/RConn1
  InternalOblique Visualization/RConn7 -- MuscleEnd27/RConn1
  Psoas Visualization/RConn1 -- MuscleEnd22/RConn1
  Psoas Visualization/LConn2 -- MuscleEnd26/RConn1
  Longissimus Visualization/RConn10 -- MuscleEnd50/RConn1
  Longissimus Visualization/LConn7 -- MuscleEnd38/RConn1
  Longissimus Visualization/LConn6 -- MuscleEnd24/RConn1
  Multifidus Visualization/RConn7 -- MuscleEnd19/RConn1
  Multifidus Visualization/RConn12 -- MuscleEnd54/RConn1
  Longissimus Visualization/LConn5 -- MuscleEnd16/RConn1
  Longissimus Visualization/RConn4 -- MuscleEnd14/RConn1
  Psoas Visualization/RConn6 -- MuscleEnd48/RConn1
  Psoas Visualization/LConn1 -- MuscleEnd25/RConn1
  RA Visualization/RConn3 -- MuscleEnd68/RConn1
  ExternalOblique Visualization/RConn7 -- MuscleEnd45/RConn1
  RA Visualization/RConn2 -- MuscleEnd47/RConn1
  Psoas Visualization/RConn7 -- MuscleEnd53/RConn1
  ExternalOblique Visualization/RConn5 -- MuscleEnd35/RConn1
  Multifidus Visualization/RConn5 -- MuscleEnd12/RConn1
  ExternalOblique Visualization/RConn6 -- MuscleEnd36/RConn1
  Longissimus Visualization/RConn8 -- MuscleEnd30/RConn1
  Multifidus Visualization/LConn4 -- MuscleEnd43/RConn1
  RA Visualization/RConn4 -- MuscleEnd67/RConn1
  Psoas Visualization/RConn2 -- MuscleEnd23/RConn1
  ExternalOblique Visualization/RConn12 -- MuscleEnd66/RConn1
  ExternalOblique Visualization/RConn9 -- MuscleEnd60/RConn1
  Multifidus Visualization/RConn3 -- MuscleEnd7/RConn1
  InternalOblique Visualization/RConn10 -- MuscleEnd34/RConn1
  Longissimus Visualization/LConn4 -- MuscleEnd10/RConn1
  Psoas Visualization/RConn4 -- MuscleEnd32/RConn1
  Longissimus Visualization/LConn2 -- MuscleEnd8/RConn1
  RA Visualization/RConn1 -- MuscleEnd42/RConn1
  Longissimus Visualization/RConn1 -- MuscleEnd3/RConn1
  Psoas Visualization/LConn3 -- R1/RConn1
  InternalOblique Visualization/RConn13 -- MuscleEnd51/RConn1
  Longissimus Visualization/RConn7 -- MuscleEnd29/RConn1
  Longissimus Visualization/RConn2 -- MuscleEnd4/RConn1
  Longissimus Visualization/RConn9 -- MuscleEnd49/RConn1
  Longissimus Visualization/RConn3 -- MuscleEnd13/RConn1
  Longissimus Visualization/RConn6 -- MuscleEnd18/RConn1
  Longissimus Visualization/LConn1 -- R/RConn1 -- Multifidus Visualization/LConn1
  Multifidus Visualization/LConn3 -- MuscleEnd6/RConn1
  Psoas Visualization/RConn3 -- MuscleEnd31/RConn1
  Psoas Visualization/RConn5 -- MuscleEnd44/RConn1
  Multifidus Visualization/RConn8 -- MuscleEnd20/RConn1
  ExternalOblique Visualization/RConn10 -- MuscleEnd63/RConn1
  ExternalOblique Visualization/RConn11 -- MuscleEnd65/RConn1
  InternalOblique Visualization/RConn17 -- MuscleEnd61/RConn1
  ExternalOblique Visualization/RConn8 -- MuscleEnd46/RConn1
  Psoas Visualization/RConn8 -- MuscleEnd56/RConn1
  Multifidus Visualization/RConn4 -- MuscleEnd11/RConn1
  Longissimus Visualization/LConn3 -- MuscleEnd9/RConn1
  InternalOblique Visualization/RConn14 -- MuscleEnd57/RConn1
  InternalOblique Visualization/RConn3 -- ExternalOblique Visualization/RConn3 -- R5/RConn1 -- ExternalOblique Visualization/RConn1 -- ExternalOblique Visualization/RConn2 -- ExternalOblique Visualization/RConn4 -- InternalOblique Visualization/RConn5 -- InternalOblique Visualization/RConn1 -- InternalOblique Visualization/RConn2 -- InternalOblique Visualization/RConn6 -- RA Visualization/LConn1 -- InternalOblique Visualization/RConn4
  Multifidus Visualization/RConn13 -- MuscleEnd58/RConn1
  Longissimus Visualization/LConn8 -- MuscleEnd52/RConn1
  Longissimus Visualization/RConn5 -- MuscleEnd17/RConn1

== system Main_C0_C3/Muscle Forces/Subsystem ==
  Muslce force : Inport
  Manual Switch1 : ManualSwitch
  Ramped : Subsystem
  Out1 : Outport
  wires:
  Manual Switch1/1 -> Out1/1
  Muslce force/1 -> Ramped/1(u), Manual Switch1/2
  Ramped/1(y) -> Manual Switch1/1

== system Main_C0_C3/Muscle Forces/Subsystem1 ==
  Muslce force : Inport
  Manual Switch1 : ManualSwitch
  Ramped : Subsystem
  Out1 : Outport
  wires:
  Manual Switch1/1 -> Out1/1
  Muslce force/1 -> Ramped/1(u), Manual Switch1/2
  Ramped/1(y) -> Manual Switch1/1

== system Main_C0_C3/Muscle Forces/Subsystem10 ==
  Muslce force : Inport
  Manual Switch1 : ManualSwitch
  Ramped : Subsystem
  Out1 : Outport
  wires:
  Manual Switch1/1 -> Out1/1
  Muslce force/1 -> Ramped/1(u), Manual Switch1/2
  Ramped/1(y) -> Manual Switch1/1

== system Main_C0_C3/Muscle Forces/Subsystem11 ==
  Muslce force : Inport
  Manual Switch1 : ManualSwitch
  Ramped : Subsystem
  Out1 : Outport
  wires:
  Manual Switch1/1 -> Out1/1
  Muslce force/1 -> Ramped/1(u), Manual Switch1/2
  Ramped/1(y) -> Manual Switch1/1

== system Main_C0_C3/Muscle Forces/Subsystem2 ==
  Muslce force : Inport
  Manual Switch1 : ManualSwitch
  Ramped : Subsystem
  Out1 : Outport
  wires:
  Manual Switch1/1 -> Out1/1
  Muslce force/1 -> Ramped/1(u), Manual Switch1/2
  Ramped/1(y) -> Manual Switch1/1

== system Main_C0_C3/Muscle Forces/Subsystem3 ==
  Muslce force : Inport
  Manual Switch1 : ManualSwitch
  Ramped : Subsystem
  Out1 : Outport
  wires:
  Manual Switch1/1 -> Out1/1
  Muslce force/1 -> Ramped/1(u), Manual Switch1/2
  Ramped/1(y) -> Manual Switch1/1

== system Main_C0_C3/Muscle Forces/Subsystem4 ==
  Muslce force : Inport
  Manual Switch1 : ManualSwitch
  Ramped : Subsystem
  Out1 : Outport
  wires:
  Manual Switch1/1 -> Out1/1
  Muslce force/1 -> Ramped/1(u), Manual Switch1/2
  Ramped/1(y) -> Manual Switch1/1

== system Main_C0_C3/Muscle Forces/Subsystem5 ==
  Muslce force : Inport
  Manual Switch1 : ManualSwitch
  Ramped : Subsystem
  Out1 : Outport
  wires:
  Manual Switch1/1 -> Out1/1
  Muslce force/1 -> Ramped/1(u), Manual Switch1/2
  Ramped/1(y) -> Manual Switch1/1

== system Main_C0_C3/Muscle Forces/Subsystem6 ==
  Muslce force : Inport
  Manual Switch1 : ManualSwitch
  Ramped : Subsystem
  Out1 : Outport
  wires:
  Manual Switch1/1 -> Out1/1
  Muslce force/1 -> Ramped/1(u), Manual Switch1/2
  Ramped/1(y) -> Manual Switch1/1

== system Main_C0_C3/Muscle Forces/Subsystem7 ==
  Muslce force : Inport
  Manual Switch1 : ManualSwitch
  Ramped : Subsystem
  Out1 : Outport
  wires:
  Manual Switch1/1 -> Out1/1
  Muslce force/1 -> Ramped/1(u), Manual Switch1/2
  Ramped/1(y) -> Manual Switch1/1

== system Main_C0_C3/Muscle Forces/Subsystem8 ==
  Muslce force : Inport
  Manual Switch1 : ManualSwitch
  Ramped : Subsystem
  Out1 : Outport
  wires:
  Manual Switch1/1 -> Out1/1
  Muslce force/1 -> Ramped/1(u), Manual Switch1/2
  Ramped/1(y) -> Manual Switch1/1

== system Main_C0_C3/Muscle Forces/Subsystem9 ==
  Muslce force : Inport
  Manual Switch1 : ManualSwitch
  Ramped : Subsystem
  Out1 : Outport
  wires:
  Manual Switch1/1 -> Out1/1
  Muslce force/1 -> Ramped/1(u), Manual Switch1/2
  Ramped/1(y) -> Manual Switch1/1
